simulink model "problem2"  (R2024b)
settings: Solver=VariableStepAuto  StartTime=0.0  StopTime=1000  RelTol=1e-6
settings Model: Creator=djd14  LastModifiedBy=djd14

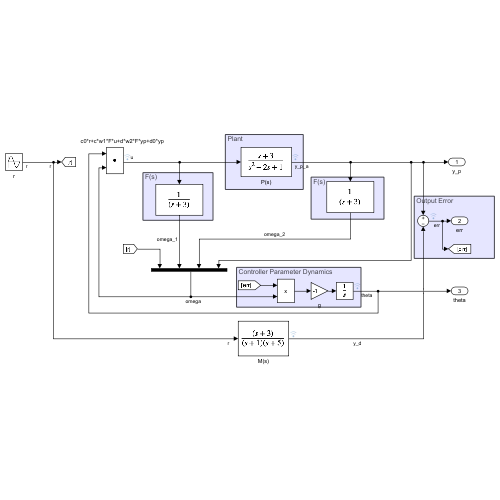
[thumbnail: Simulink's stored preview of the top-level diagram]
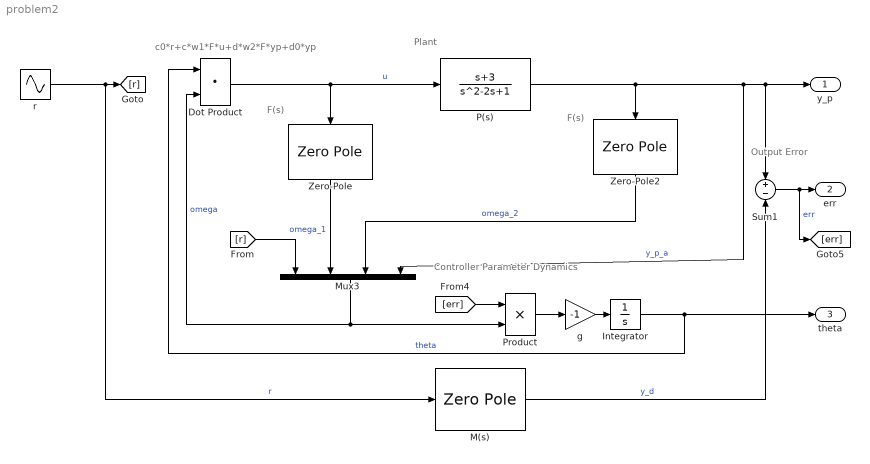
== system problem2 ==
  note: Output Error
  note: c0*r+c*w1*F*u+d*w2*F*yp+d0*yp
  note: Plant
  note: Controller Parameter Dynamics
  note: F(s)
  note: F(s)
  Dot Product : DotProduct  OutDataTypeStr=Inherit: Inherit via internal rule
  Integrator : Integrator
  M(s) : ZeroPole  Zeros=[-3]  Poles=[-1 -5]  Gain=1
  Mux3 : Mux
  P(s) : TransferFcn  Numerator=[1 3]  Denominator=[1 -2 1]
  Product : Product
  Sum1 : Sum  Inputs=+|-
  Zero-Pole : ZeroPole  Zeros=[]  Poles=[-3]  Gain=1
  Zero-Pole2 : ZeroPole  Zeros=[]  Poles=[-3]  Gain=1
  g : Gain  Gain=-1
  r : Sin  Amplitude=2  SampleTime=0
  y_p : Outport
  err : Outport  Port=2
  theta : Outport  Port=3
  wires:
  M(s)/1 -> Sum1/2  "y_d"
  Sum1/1 -> [err], err/1  "err"
  Zero-Pole/1 -> Mux3/2  "omega_1"
  Zero-Pole2/1 -> Mux3/3  "omega_2"
  g/1 -> Integrator/1
  Product/1 -> g/1
  [err] -> Product/1
  Integrator/1 -> Dot Product/1, theta/1  "theta"
  Dot Product/1 -> Zero-Pole/1, P(s)/1  "u"
  Mux3/1 -> Dot Product/2, Product/2  "omega"
  [r] -> Mux3/1
  P(s)/1 -> Mux3/4, Sum1/1, y_p/1, Zero-Pole2/1  "y_p_a"
  r/1 -> M(s)/1, [r]  "r"
